simulink model "Level5"  (R2012b)
settings: Solver=FixedStepDiscrete  StartTime=0.0  StopTime=50  RelTol=1e-3
InitFcn:
  | N=256;
  | Fs = 1000;
  | bw = 5.6;
undefined symbols (not defined in the file): gcbh, rmidispblock
settings Model: RequirementInfo={'other' '..\..\..\requirements\ebd_srs.doc' '@Simulink_requirement_level5' 'true' '3.1.3.6 Level 5 PD' 'Requirement' } %GIDa_89a39d40_ab35_46b7_b86d_85f19b3a7739  Creator=aanantha  LastModifiedBy=klindqvi
settings DataIOCC: SaveFormat=Structure  SignalLoggingSaveFormat=ModelDataLogs  SaveOutput=off  SaveTime=off  SignalLoggingName=logsOut
settings OptimizationCC: InlineParams=on  OptimizeModelRefInitCode=on  LifeSpan=1
settings DebuggingCC: ReadBeforeWriteMsg=DisableAll  WriteAfterWriteMsg=DisableAll  WriteAfterReadMsg=DisableAll  SolverPrmCheckMsg=none  InheritedTsInSrcMsg=none  ParameterPrecisionLossMsg=none  FcnCallInpInsideContextMsg=EnableAllAsWarning
settings HardwareCC: ProdLargestAtomicInteger=Long  ProdLargestAtomicFloat=Double  ProdEndianess=LittleEndian  ProdHWDeviceType=ARM Compatible->ARM Cortex
settings RTWCC: SystemTargetFile=ert.tlc  TemplateMakefile=ert_default_tmf  Description=Embedded Coder  GenerateReport=on  RTWVerbose=off  ProcessScript=ert_make_rtw_hook  IncludeHyperlinkInReport=on  LaunchReport=on  PortableWordSizes=on  CodeProfilingSaveOptions=AllData  GenerateTraceInfo=on  GenerateTraceReportSl=on  GenerateTraceReportSf=on  GenerateTraceReportEml=on  GenerateCodeMetricsReport=on
settings CodeAppCC: IgnoreCustomStorageClasses=off
settings ERTTargetCC: CodeReplacementLibrary=GCC ARM Cortex-A8  MultiwordLength=2048  GenerateSampleERTMain=on  ERTCustomFileTemplate=example_file_process.tlc  ConvertIfToSwitch=off  SuppressUnreachableDefaultCases=off

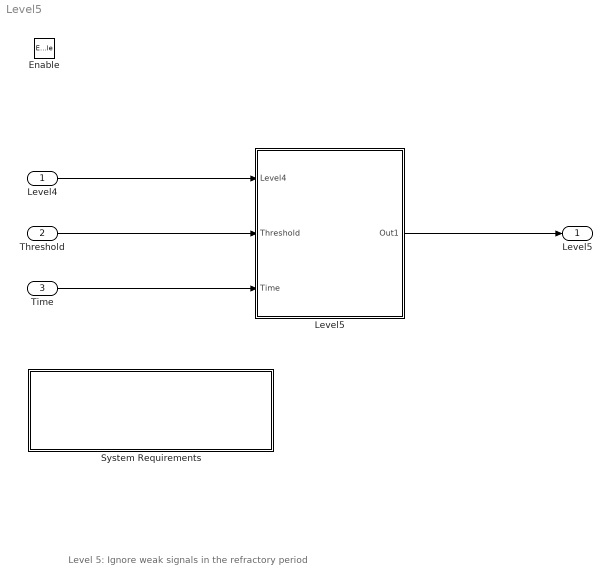
== system Level5 ==
  note: Level 5:
      | Ignore weak signals in the refractory period
  Level4 : Inport  OutDataTypeStr=double  PortDimensions=1  SampleTime=[0.08900000000000001,0]
  Threshold : Inport  Port=2  OutDataTypeStr=double  PortDimensions=1  SampleTime=[0.08900000000000001,0]
  Time : Inport  Port=3  OutDataTypeStr=uint32  PortDimensions=1  SampleTime=[0.08900000000000001,0]
  Enable : EnablePort  SampleTime=[0.08900000000000001,0]  OutDataTypeStr=boolean
  "Level5 " : Subsystem
  System Requirements : Subsystem  LoadFcn=rmidispblock('load',gcbh)  mask(System Requirements){id=SystemReq, title=System Requirements}
      mask prompts: title "Block Title"
      mask help: Lists the requirements for the current model.
      mask init:
      | id = 'SystemReq';
      | [w,h] = rmidispblock('display',gcbh);
      settings: CopyFcn=rmidispblock('create',gcbh)  DeleteFcn=rmidispblock('delete',gcbh)  ModelCloseFcn=rmidispblock('close',gcbh)  PreSaveFcn=rmidispblock('close',gcbh)  PostSaveFcn=rmidispblock('open',gcbh)  OpenFcn=rmidispblock('open',gcbh)  MoveFcn=rmidispblock('move',gcbh)
      mask Help: helpview(fullfile(docroot,'toolbox','slvnv','slvnv.map'),'systemrequirements')
      mask Display: text(w/2,h-4,rmidispblock('title',gcbh),'horizontalAlignment','center','verticalAlignment','top')
  Level5 : Outport  OutDataTypeStr=boolean  PortDimensions=1  SampleTime=[0.08900000000000001,0]  OutputWhenDisabled=reset  InitialOutput=false
  wires:
  Level4/1 -> "Level5 "/1(Level4)
  Threshold/1 -> "Level5 "/2(Threshold)
  Time/1 -> "Level5 "/3(Time)
  "Level5 "/1(Out1) -> Level5/1

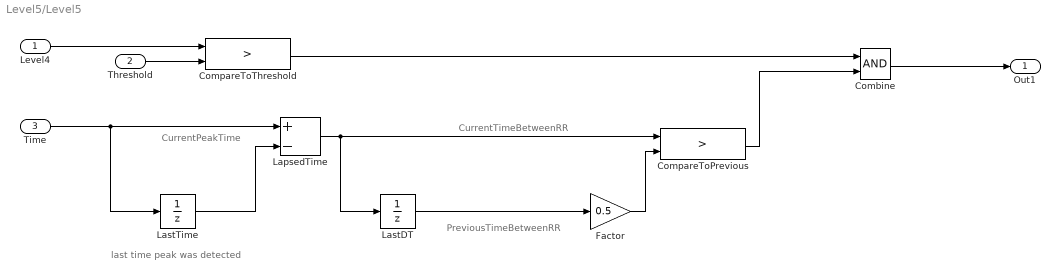
== system Level5/Level5  ==
  note: CurrentTimeBetweenRR
  note: last time peak was detected
  note: CurrentPeakTime
  note: PreviousTimeBetweenRR
  Level4 : Inport
  Threshold : Inport  Port=2  OutDataTypeStr=double  PortDimensions=1  SampleTime=[0.08900000000000001,0]
  Time : Inport  Port=3
  Combine : Logic  AllPortsSameDT=off  OutDataTypeStr=boolean
  CompareToPrevious : RelationalOperator  Operator=>  OutDataTypeStr=boolean
  CompareToThreshold : RelationalOperator  Operator=>  OutDataTypeStr=boolean
  Factor : Gain  Gain=0.5
  LapsedTime : Sum  Inputs=+-
  LastDT : UnitDelay  SampleTime=-1
  LastTime : UnitDelay  SampleTime=-1
  Out1 : Outport
  wires:
  Time/1 -> LastTime/1, LapsedTime/1
  CompareToThreshold/1 -> Combine/1
  LapsedTime/1 -> LastDT/1, CompareToPrevious/1
  Factor/1 -> CompareToPrevious/2
  LastDT/1 -> Factor/1
  Threshold/1 -> CompareToThreshold/2
  LastTime/1 -> LapsedTime/2
  CompareToPrevious/1 -> Combine/2
  Combine/1 -> Out1/1
  Level4/1 -> CompareToThreshold/1

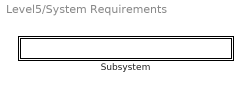
== system Level5/System Requirements ==
  Subsystem : Subsystem  mask{label=0, index=1}
      mask init:
      | label = rmidispblock('label',index);
      settings: OpenFcn=rmidispblock('openReq',gcbh);
      mask Display: text(0,0,label,'horizontalAlignment','left','verticalAlignment','bottom')

== system Level5/System Requirements/Subsystem ==
